simulink model "Ex1_model"  (R2024b)
settings: Solver=VariableStepAuto  StartTime=0.0  StopTime=10.0  RelTol=1e-3
values from neighbouring files (symbols this model uses):
  A = [0, 1; 0, -10]    [Ex1_script.m]    (also in Ex3_script.m = [0, 1; -2, -40]; Ex4_script.m = [0,1; 0,-20])
  B = [0; 120]    [Ex1_script.m]    (also in Ex3_script.m = [0; 40]; Ex4_script.m = [0; 60])
  C = [1, 0]    [Ex1_script.m]    (also in Ex3_script.m; Ex4_script.m)
  D = 0    [Ex1_script.m]    (also in Ex3_script.m; Ex4_script.m)
  Kd = Kp*Td    [Ex1_script.m]
  Ki = Kp/Ti    [Ex1_script.m]    (also in Ex2_script.m = Ke(1); Ex3_script.m = Ke(1))
  Kp = dK*cos(dphi)    [Ex1_script.m]
  Kw = 5/ts    [Ex1_script.m]
  Tl = 1/(tau*wgc)    (= 0.0277777777778)    [Ex1_script.m]
libraries: simulink x1
settings Model: Creator=pries  LastModifiedBy=pries

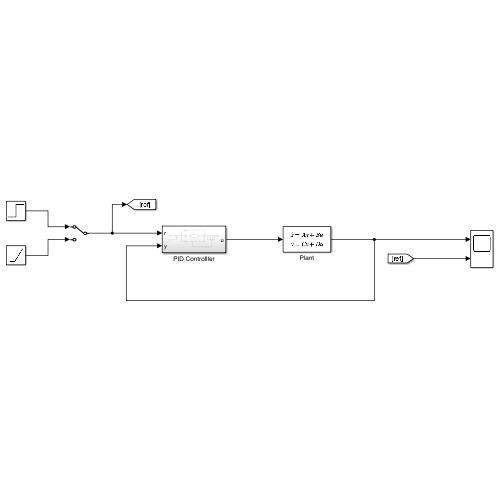
[thumbnail: Simulink's stored preview of the top-level diagram]
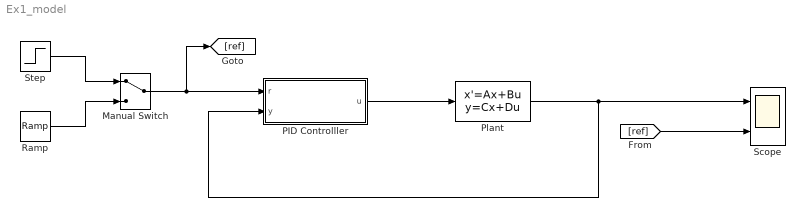
== system Ex1_model ==
  Manual Switch : ManualSwitch
  PID Controlller : Subsystem
  Plant : StateSpace  A=A  B=B  C=C  D=D  InitialCondition=0
  Ramp : simulink/Sources/Ramp  slope=30  start=0  InitialOutput=0
  Scope : Scope  NumInputPorts=2
  Step : Step  Time=0  SampleTime=0
  wires:
  PID Controlller/1(u) -> Plant/1
  Plant/1 -> Scope/1, PID Controlller/2(y)
  Manual Switch/1 -> [ref], PID Controlller/1(r)
  Step/1 -> Manual Switch/1
  Ramp/1 -> Manual Switch/2
  [ref] -> Scope/2

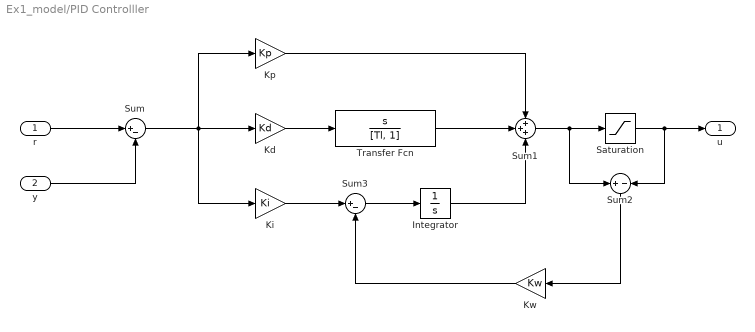
== system Ex1_model/PID Controlller ==
  r : Inport
  y : Inport  Port=2
  Integrator : Integrator
  Kd : Gain  Gain=Kd
  Ki : Gain  Gain=Ki
  Kp : Gain  Gain=Kp
  Kw : Gain  Gain=Kw
  Saturation : Saturate  UpperLimit=10  LowerLimit=-10
  Sum : Sum  Inputs=|+-
  Sum1 : Sum  Inputs=+++
  Sum2 : Sum  Inputs=+|-
  Sum3 : Sum  Inputs=|+-
  Transfer Fcn : TransferFcn  Numerator=[1,0]  Denominator=[Tl, 1]
  u : Outport
  wires:
  r/1 -> Sum/1
  Sum/1 -> Ki/1, Kp/1, Kd/1
  y/1 -> Sum/2
  Kd/1 -> Transfer Fcn/1
  Kp/1 -> Sum1/1
  Transfer Fcn/1 -> Sum1/2
  Integrator/1 -> Sum1/3
  Sum1/1 -> Sum2/1, Saturation/1
  Saturation/1 -> Sum2/2, u/1
  Ki/1 -> Sum3/1
  Sum3/1 -> Integrator/1
  Kw/1 -> Sum3/2
  Sum2/1 -> Kw/1
